simulink model "porte_avion_sym"  (R2025a)
settings: Solver=VariableStepAuto  StartTime=0.0  StopTime=20.0  RelTol=1e-3
values from neighbouring files (symbols this model uses):
  A = [0    1  0    0 ... (first row only)    [porte_avion.m]
  B = [0 ... (first row only)    [porte_avion.m]
  C = [1 0 0 0 ... (first row only)    [porte_avion.m]
  D = [0 ... (first row only)    [porte_avion.m]
  theta_0 = pi/3    (= 1.0471975512)    [porte_avion.m]
  theta_dot_0 = 0    [porte_avion.m]
  X_0 = [x_0 ... (first row only)    [porte_avion.m]
  x_0 = 0    [porte_avion.m]
  x_dot_0 = 0    [porte_avion.m]
settings Model: Creator=vikfo  LastModifiedBy=vikfo

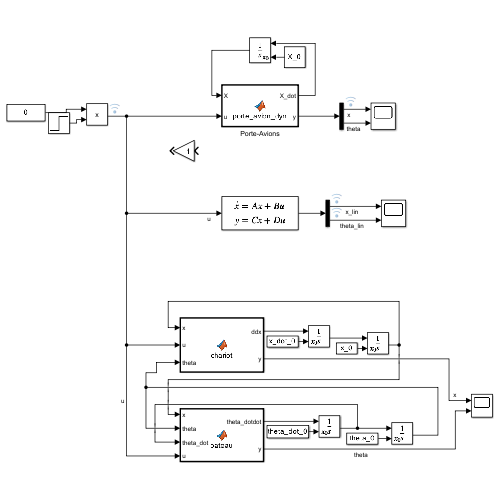
[thumbnail: Simulink's stored preview of the top-level diagram]
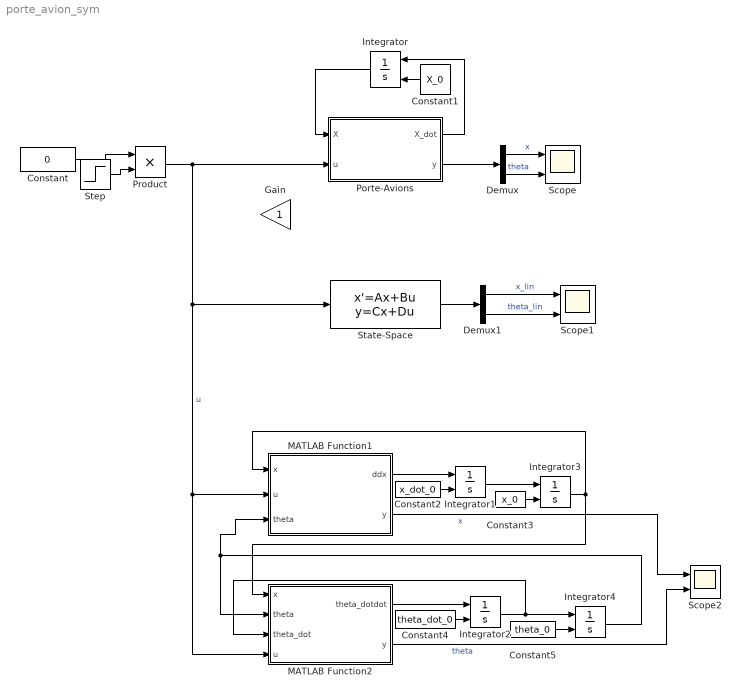
== system porte_avion_sym ==
  Constant : Constant  Value=0
  Constant1 : Constant  Value=X_0
  Constant2 : Constant  Value=x_dot_0
  Constant3 : Constant  Value=x_0
  Constant4 : Constant  Value=theta_dot_0
  Constant5 : Constant  Value=theta_0
  Demux : Demux  Outputs=2
  Demux1 : Demux  Outputs=2
  Gain : Gain
  Integrator{,1..4} (5 alike) : Integrator  InitialConditionSource=external
  MATLAB Function1 : MATLAB Function  TreatAsAtomicUnit=on
  MATLAB Function2 : MATLAB Function  TreatAsAtomicUnit=on
  Porte-Avions : MATLAB Function  TreatAsAtomicUnit=on
  Product : Product
  Scope : Scope  NumInputPorts=2
      settings: ActiveDisplayYMinimum=-1.2564751864895671  ActiveDisplayYMaximum=11.261238610356225
  Scope1 : Scope  NumInputPorts=2
      settings: ActiveDisplayYMinimum=-1  ActiveDisplayYMaximum=1
  Scope2 : Scope  NumInputPorts=2
      settings: ActiveDisplayYMinimum=-1  ActiveDisplayYMaximum=1  DataLoggingVariableName=ScopeData2
  State-Space : StateSpace  A=A  B=B  C=C  D=D  InitialCondition=X_0
  Step : Step  Time=2  SampleTime=0
  wires:
  Porte-Avions/1(X_dot) -> Integrator/1
  Integrator/1 -> Porte-Avions/1(X)
  Step/1 -> Product/2
  Constant/1 -> Product/1
  Product/1 -> MATLAB Function2/4(u), MATLAB Function1/2(u), State-Space/1, Porte-Avions/2(u)  "u"
  Demux/2 -> Scope/2  "theta"
  Constant1/1 -> Integrator/2
  Porte-Avions/2(y) -> Demux/1
  Demux/1 -> Scope/1  "x"
  Demux1/2 -> Scope1/2  "theta_lin"
  Demux1/1 -> Scope1/1  "x_lin"
  State-Space/1 -> Demux1/1
  MATLAB Function1/1(ddx) -> Integrator1/1
  MATLAB Function2/1(theta_dotdot) -> Integrator2/1
  Integrator1/1 -> Integrator3/1
  Integrator3/1 -> MATLAB Function1/1(x), MATLAB Function2/1(x)
  Integrator2/1 -> MATLAB Function2/3(theta_dot), Integrator4/1
  Integrator4/1 -> MATLAB Function1/3(theta), MATLAB Function2/2(theta)
  MATLAB Function2/2(y) -> Scope2/2  "theta"
  MATLAB Function1/2(y) -> Scope2/1  "x"
  Constant2/1 -> Integrator1/2
  Constant3/1 -> Integrator3/2
  Constant4/1 -> Integrator2/2
  Constant5/1 -> Integrator4/2

== matlab function porte_avion_sym/MATLAB Function1 ==
  data: ddx output; x input; y output; u input; theta input
function [ddx, y]  = chariot(x, u, theta)
g = 9.81;
a = 250e3;

ddx = - g * sin(theta) + (1/a) * u;
y = x;

== matlab function porte_avion_sym/Porte-Avions ==
  data: X input; u input; X_dot output; y output
function [X_dot, y]= porte_avion_dyn(X, u)
    g = 9.81;
    a = 250e3;
    b = 1e9;
    c = 0.4e9;
    d = 500e6;
    e = 250e3;
    f = 60;

    x         = X(1);
    x_dot     = X(2);
    theta     = X(3);
    theta_dot = X(4);

    X_dot = zeros(4,1);

    % Équations d'état
    X_dot(1) = x_dot;
    X_dot(2) = - g * sin(theta) + (1/a) * u;
    X_dot(3) = theta_dot;
    X_dot(4) = - (e/b) * cos(theta) * x - (d/b) * sin(theta) - (c/b) * theta_dot + (f/b) * u;
    
    y = zeros(2,1);
    y(1) = x;
    y(2) = theta;

end

== matlab function porte_avion_sym/MATLAB Function2 ==
  data: x input; theta_dotdot output; theta input; theta_dot input; u input; y output
function [theta_dotdot, y] = bateau(x, theta, theta_dot, u)
b = 1e9;
c = 0.4e9;
d = 500e6;
e = 250e3;
f = 60;

theta_dotdot = - (e/b) * cos(theta) * x - (d/b) * sin(theta) - (c/b) * theta_dot + (f/b) * u;
y = theta;
